simulink model "PositionControl"  (R2020a)
settings: Solver=VariableStepAuto  StartTime=0.0  StopTime=10.0  RelTol=1e-3
settings Model: Creator=Acer  LastModifiedBy=Acer

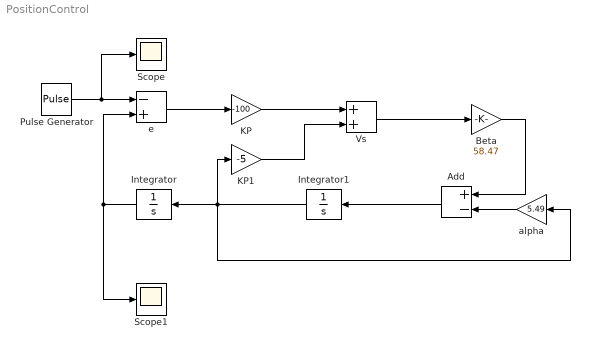
== system PositionControl ==
  Add : Sum  Inputs=+-
  Beta : Gain  Gain=58.47
  Integrator : Integrator
  Integrator1 : Integrator
  KP : Gain  Gain=-100
  KP1 : Gain  Gain=-5
  Pulse Generator : DiscretePulseGenerator  PulseType=Time based  Amplitude=5  Period=5  PulseWidth=50
  Scope : Scope
  Scope1 : Scope
  Vs : Sum
  alpha : Gain  Gain=5.49
  e : Sum  Inputs=-+
  wires:
  Pulse Generator/1 -> Scope/1, e/1
  e/1 -> KP/1
  Integrator/1 -> e/2, Scope1/1
  Integrator1/1 -> alpha/1, KP1/1, Integrator/1
  KP/1 -> Vs/1
  KP1/1 -> Vs/2
  Vs/1 -> Beta/1
  Add/1 -> Integrator1/1
  Beta/1 -> Add/1
  alpha/1 -> Add/2
